simulink model "EggBoilingSimulator"  (R2019b)
settings: Solver=VariableStepAuto  StartTime=0.0  StopTime=10.0  RelTol=1e-3
libraries: fuzblock x1
settings Model: Creator=ASUS  LastModifiedBy=ASUS

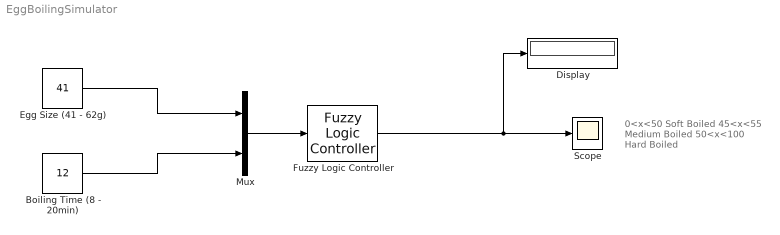
== system EggBoilingSimulator ==
  note: 0<x<50     Soft Boiled
      |  45<x<55    Medium Boiled
      | 50<x<100   Hard Boiled
  Boiling Time (8 - 20min) : Constant  Value=12  OutMin=[8]  OutMax=[20]
  Display : Display
  Egg Size (41 - 62g) : Constant  Value=41  OutMin=[41]  OutMax=[61]
  Fuzzy Logic Controller : fuzblock/Fuzzy Logic  Controller  FIS='FuzzyProjectYeni.fis'  OutputSampleNumber=101  DataType=double  FuzzifiedInputs=off  RuleFiringStrengths=off  RuleOutputs=off  AggregatedOutputs=off  SimulateUsing=Interpreted execution  OutOfRangeInputValueMessage=warning  NoRuleFiredMessage=warning  EmptyOutputFuzzySetMessage=warning
  Mux : Mux  Inputs=2
  Scope : Scope
  wires:
  Egg Size (41 - 62g)/1 -> Mux/1
  Boiling Time (8 - 20min)/1 -> Mux/2
  Mux/1 -> Fuzzy Logic Controller/1
  Fuzzy Logic Controller/1 -> Scope/1, Display/1
